simulink model "P2_3a"  (R2014a)
settings: Solver=ode45  StartTime=0.0  StopTime=200  RelTol=1e-3
settings Model: Creator=Jhonantans  LastModifiedBy=Jhonantans

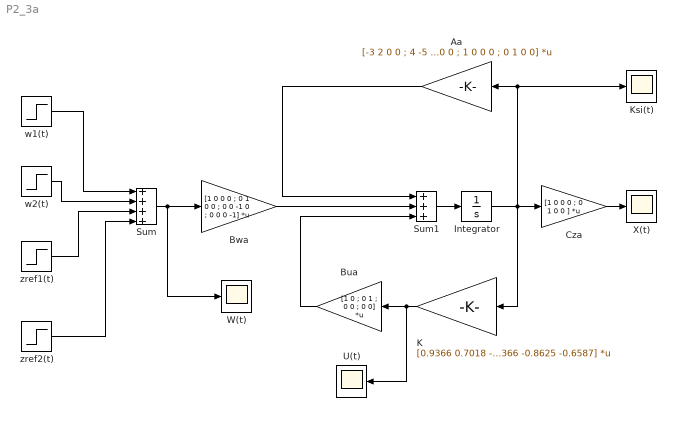
== system P2_3a ==
  Aa : Gain  Gain=[-3 2 0 0 ; 4 -5 0 0 ; 1 0 0 0 ; 0 1 0 0]  Multiplication=Matrix(K*u) (u vector)
  Bua : Gain  Gain=[1 0 ; 0 1 ; 0 0 ; 0 0]  Multiplication=Matrix(K*u) (u vector)
  Bwa : Gain  Gain=[1 0 0 0 ; 0 1 0 0 ; 0 0 -1 0 ; 0 0 0 -1]  Multiplication=Matrix(K*u) (u vector)
  Cza : Gain  Gain=[1 0 0 0 ; 0 1 0 0 ]  Multiplication=Matrix(K*u) (u vector)
  Integrator : Integrator
  K : Gain  Gain=[0.9366 0.7018 -0.6587 0.8625; -6.7018 2.9366 -0.8625 -0.6587]  Multiplication=Matrix(K*u) (u vector)
  Ksi(t) : Scope
      settings: SaveName=ScopeData3
  Sum : Sum  Inputs=++++
  Sum1 : Sum  Inputs=+++
  U(t) : Scope
      settings: SaveName=ScopeData2
  W(t) : Scope
      settings: TimeRange=200  YMin=-4000  YMax=1000
  X(t) : Scope
  w1(t) : Step  Time=125  Before=[1; 0; 0; 0]  After=[2; 0; 0; 0]  SampleTime=0
  w2(t) : Step  Time=100  Before=[0; 2; 0; 0]  After=[0; 3; 0; 0]  SampleTime=0
  zref1(t) : Step  Time=75  Before=[0; 0; 4; 0]  After=[0; 0; 6; 0]  SampleTime=0
  zref2(t) : Step  Time=50  Before=[0; 0; 0; 5]  After=[0; 0; 0; 8]  SampleTime=0
  wires:
  Integrator/1 -> Aa/1, Ksi(t)/1, K/1, Cza/1
  Aa/1 -> Sum1/1
  Bwa/1 -> Sum1/2
  Bua/1 -> Sum1/3
  K/1 -> Bua/1, U(t)/1
  Sum1/1 -> Integrator/1
  Cza/1 -> X(t)/1
  w1(t)/1 -> Sum/1
  w2(t)/1 -> Sum/2
  zref2(t)/1 -> Sum/4
  zref1(t)/1 -> Sum/3
  Sum/1 -> W(t)/1, Bwa/1
